simulink model "Simulation_6DOFTesting"  (R2024a)
settings: Solver=ode4  StartTime=initial_time  StopTime=final_time  FixedStep=timestep  RelTol=1e-3
values from neighbouring files (symbols this model uses):
  aEarth = 0    [CodeTesting_6DOF.m]    (also in Constants_6DOF.m = 6378137; Constants_6DOFTesting.m = 6378137)
  alphaArray = [-30, -25, -20, -15, -10, -5, 0, 5, 10, 15, 20, 25, 30]    [CodeTesting_6DOF.m]    (also in Constants_6DOF.m; Constants_6DOFTesting.m)
  altitudeArray = [0, 1000, 2000, 3000, 4000, 5000, 6000, 7000, 8000, 9000, 10000, 15000, 20000,      25000, 30000, 35000, 40000, 45000, 50000, 55000, 60000]    [CodeTesting_6DOF.m]    (also in Constants_6DOF.m; Constants_6DOFTesting.m)
  bEarth = 0    [CodeTesting_6DOF.m]    (also in Constants_6DOF.m = 6356752.3; Constants_6DOFTesting.m = 6356752.3)
  cD_3DArray = zeros(numAoAs, numMachs, numAltitudes)    [CodeTesting_6DOF.m]    (also in Constants_6DOF.m; Constants_6DOFTesting.m)
  cL_3DArray = zeros(numAoAs, numMachs, numAltitudes)    [CodeTesting_6DOF.m]    (also in Constants_6DOF.m; Constants_6DOFTesting.m)
  densityList = rhoList    [CodeTesting_6DOF.m]    (also in Constants_6DOF.m = usAtmosphere.x_; Constants_6DOFTesting.m = usAtmosphere.x_)
  height0 = 0    [Constants_6DOF.m]    (also in Constants_6DOFTesting.m = 5000)
  heightsList = usAtmosphere.Z    [CodeTesting_6DOF.m]    (also in Constants_6DOF.m; Constants_6DOFTesting.m)
  inertialPitch0 = deg2rad(inertialPitch0)    [Constants_6DOFTesting.m]
  inertialRoll0 = deg2rad(inertialRoll0)    [Constants_6DOFTesting.m]
  inertialYaw0 = deg2rad(inertialYaw0)    [Constants_6DOFTesting.m]
  Ixx = 10    [CodeTesting_6DOF.m]    (also in Constants_6DOF.m; Constants_6DOFTesting.m = 4.88094462)
  Ixz = 10    [CodeTesting_6DOF.m]    (also in Constants_6DOF.m = 1; Constants_6DOFTesting.m = 4.88094462)
  Iyy = 10    [CodeTesting_6DOF.m]    (also in Constants_6DOF.m; Constants_6DOFTesting.m = 4.88094462)
  Izz = 10    [CodeTesting_6DOF.m]    (also in Constants_6DOF.m; Constants_6DOFTesting.m = 4.88094462)
  latitude0 = pi/4    (= 0.785398163397)    [CodeTesting_6DOF.m]    (also in Constants_6DOF.m = deg2rad(latitude0); Constants_6DOFTesting.m = deg2rad(latitude0))
  longitude0 = pi/4    (= 0.785398163397)    [CodeTesting_6DOF.m]    (also in Constants_6DOF.m = deg2rad(longitude0); Constants_6DOFTesting.m = deg2rad(longitude0))
  m0 = 10    [CodeTesting_6DOF.m]    (also in Constants_6DOF.m = 50; Constants_6DOFTesting.m = 14.5939029)
  machArray = [0.5, 1.0, 1.5, 2.0, 2.5, 3.0, 3.5, 4.0, 4.5, 5.0, 5.5, 6.0, 6.5, 7.0, 7.5, 8.0,      8.5, 9.0, 9.5, 10.0]    [CodeTesting_6DOF.m]    (also in Constants_6DOF.m; Constants_6DOFTesting.m)
  omegaEarth = omega_earth    (= 7.2921159e-05)    [CodeTesting_6DOF.m]    (also in Constants_6DOF.m; Constants_6DOFTesting.m)
  p0Body = deg2rad(p0Body)    [Constants_6DOFTesting.m]
  phiBody0 = deg2rad(phiBody0)    [Constants_6DOFTesting.m]
  psiBody0 = deg2rad(psiBody0)    [Constants_6DOFTesting.m]
  q0Body = deg2rad(q0Body)    [Constants_6DOFTesting.m]
  r0Body = deg2rad(r0Body)    [Constants_6DOFTesting.m]
  rEarth = r_earth    (= 6371008.8)    [CodeTesting_6DOF.m]    (also in Constants_6DOF.m; Constants_6DOFTesting.m)
  temperatureList = usAtmosphere.T    [CodeTesting_6DOF.m]    (also in Constants_6DOF.m; Constants_6DOFTesting.m)
  thetaBody0 = deg2rad(thetaBody0)    [Constants_6DOFTesting.m]
  u0Body = 304.8    [Constants_6DOFTesting.m]
  v0Body = 0    [Constants_6DOFTesting.m]
  w0Body = -1 * w0Body    (= 0)    [Constants_6DOFTesting.m]
  wingArea = 0    [CodeTesting_6DOF.m]    (also in Constants_6DOF.m = 50; Constants_6DOFTesting.m = 0.09290304)
undefined symbols (not defined in the file or in its folder): inertialX0, inertialY0, inertialZ0
libraries: simulink_extras x18
(part 1 of 2)
settings Model: Creator=641893  LastModifiedBy=641893

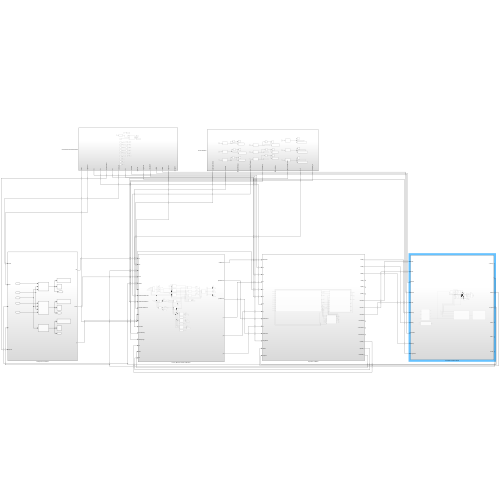
[thumbnail: Simulink's stored preview of the top-level diagram]
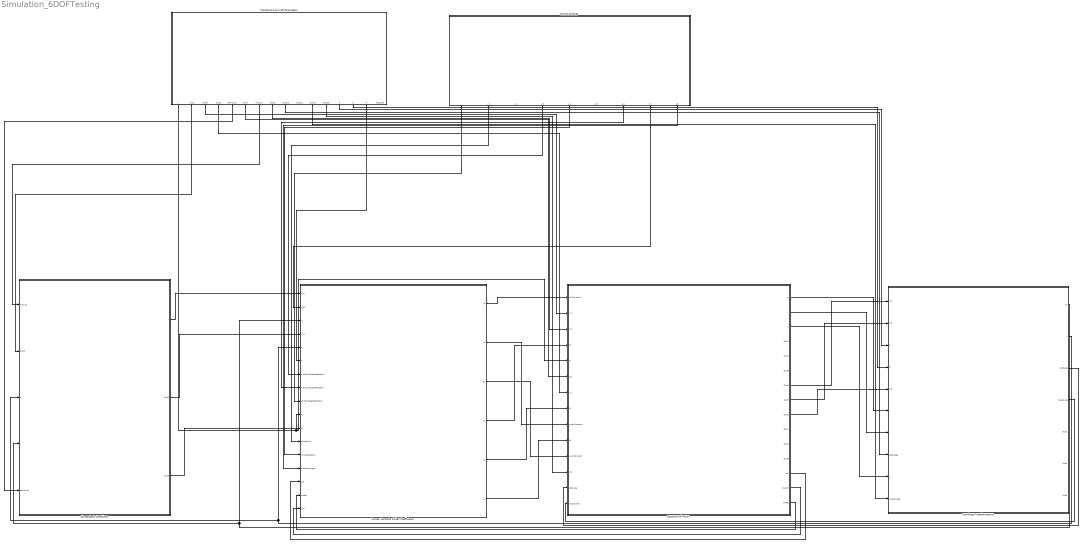
== system Simulation_6DOFTesting ==
  Atmospheric Conditions : Subsystem
  Constants & Aircraft Parameters : Subsystem
  Control Surfaces : Subsystem
  Coordinate Transformations : Subsystem
  Equations of Motion : Subsystem
  "Forces, Moments & their Coefficients" : Subsystem
  wires:
  Atmospheric Conditions/1(y) -> "Forces, Moments & their Coefficients"/1(rho)
  Atmospheric Conditions/2(Out2) -> "Forces, Moments & their Coefficients"/4(In4)
  Atmospheric Conditions/3(Out3) -> "Forces, Moments & their Coefficients"/11(g)
  Constants & Aircraft Parameters/7(rhoList) -> Atmospheric Conditions/1(rhoList)
  Constants & Aircraft Parameters/2(hList) -> Atmospheric Conditions/2(hList)
  Constants & Aircraft Parameters/5(tempList) -> Atmospheric Conditions/5(tempList)
  Coordinate Transformations/1(y4) -> "Forces, Moments & their Coefficients"/3(v), Atmospheric Conditions/4(v)
  Coordinate Transformations/2(y) -> "Forces, Moments & their Coefficients"/5(y), Atmospheric Conditions/3(r)
  Constants & Aircraft Parameters/15(A) -> "Forces, Moments & their Coefficients"/6(A)
  Constants & Aircraft Parameters/1(y) -> Equations of Motion/5(m), "Forces, Moments & their Coefficients"/10(m)
  Control Surfaces/1(y) -> "Forces, Moments & their Coefficients"/9(rollSurfaceDeflection)
  Control Surfaces/4(y3) -> "Forces, Moments & their Coefficients"/7(pitchSurfaceDeflection)
  Control Surfaces/7(y6) -> "Forces, Moments & their Coefficients"/8(yawSurfaceDeflection)
  Control Surfaces/2(y1) -> "Forces, Moments & their Coefficients"/12(thrustAoA)
  Control Surfaces/5(y4) -> "Forces, Moments & their Coefficients"/13(thrustSideslip)
  "Forces, Moments & their Coefficients"/1(y5) -> Equations of Motion/1(rollMoment)
  "Forces, Moments & their Coefficients"/2(y8) -> Equations of Motion/9(pitchMoment)
  "Forces, Moments & their Coefficients"/3(y11) -> Equations of Motion/11(yawMoment)
  "Forces, Moments & their Coefficients"/6(y3) -> Equations of Motion/10(Fz)
  "Forces, Moments & their Coefficients"/5(y2) -> Equations of Motion/8(Fy)
  "Forces, Moments & their Coefficients"/4(y1) -> Equations of Motion/4(Fx)
  Constants & Aircraft Parameters/3(Out4) -> Equations of Motion/2(Ixx)
  Constants & Aircraft Parameters/4(Out5) -> Equations of Motion/7(Iyy)
  Constants & Aircraft Parameters/6(Out7) -> Equations of Motion/6(Izz)
  Constants & Aircraft Parameters/8(Out9) -> Equations of Motion/3(Ixz)
  Equations of Motion/1(u) -> Coordinate Transformations/6(u)
  Equations of Motion/2(v) -> Coordinate Transformations/7(v)
  Equations of Motion/3(w) -> Coordinate Transformations/9(w)
  Constants & Aircraft Parameters/9(Out10) -> Coordinate Transformations/8(latitude0)
  Constants & Aircraft Parameters/13(a) -> Coordinate Transformations/3(a)
  Constants & Aircraft Parameters/14(b) -> Coordinate Transformations/4(b)
  Constants & Aircraft Parameters/11(Out12) -> Coordinate Transformations/10(longitude0)
  Equations of Motion/7(Out4) -> Coordinate Transformations/1(In1)
  Equations of Motion/8(Out5) -> Coordinate Transformations/2(In3)
  Equations of Motion/9(Out6) -> Coordinate Transformations/5(In8)
  Control Surfaces/8(y7) -> "Forces, Moments & their Coefficients"/2(AoA)
  Control Surfaces/9(y8) -> "Forces, Moments & their Coefficients"/14(sideslipAngle)
  Equations of Motion/13(phi) -> "Forces, Moments & their Coefficients"/15(psi)
  Equations of Motion/15(theta) -> "Forces, Moments & their Coefficients"/16(theta)
  Equations of Motion/14(Out10) -> "Forces, Moments & their Coefficients"/17(phi)
  Constants & Aircraft Parameters/12(Out13) -> Equations of Motion/12(In1)
  Coordinate Transformations/3(latitude) -> Equations of Motion/13(latitude)
  Coordinate Transformations/4(longitude) -> Equations of Motion/14(longitude)

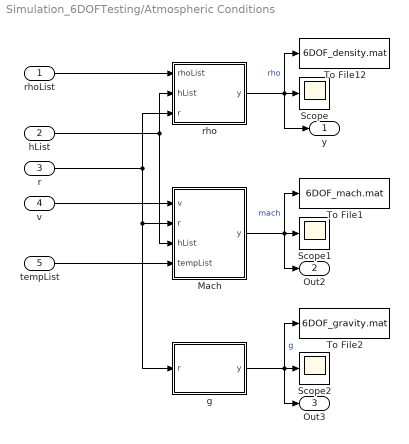
== system Simulation_6DOFTesting/Atmospheric Conditions ==
  rhoList : Inport
  hList : Inport  Port=2
  r : Inport  Port=3
  v : Inport  Port=4
  tempList : Inport  Port=5
  Mach : MATLAB Function  TreatAsAtomicUnit=on
  Scope : Scope
  Scope1 : Scope
  Scope2 : Scope
  To File1 : ToFile  Filename=6DOF_mach.mat
  To File12 : ToFile  Filename=6DOF_density.mat
  To File2 : ToFile  Filename=6DOF_gravity.mat
  g : MATLAB Function  TreatAsAtomicUnit=on
  rho : MATLAB Function  TreatAsAtomicUnit=on
  y : Outport
  Out2 : Outport  Port=2
  Out3 : Outport  Port=3
  wires:
  rho/1(y) -> Scope/1, To File12/1, y/1  "rho"
  Mach/1(y) -> Scope1/1, To File1/1, Out2/1  "mach"
  g/1(y) -> To File2/1, Scope2/1, Out3/1  "g"
  hList/1 -> rho/2(hList), Mach/3(hList)
  v/1 -> Mach/1(v)
  tempList/1 -> Mach/4(tempList)
  r/1 -> rho/3(r), g/1(r), Mach/2(r)
  rhoList/1 -> rho/1(rhoList)

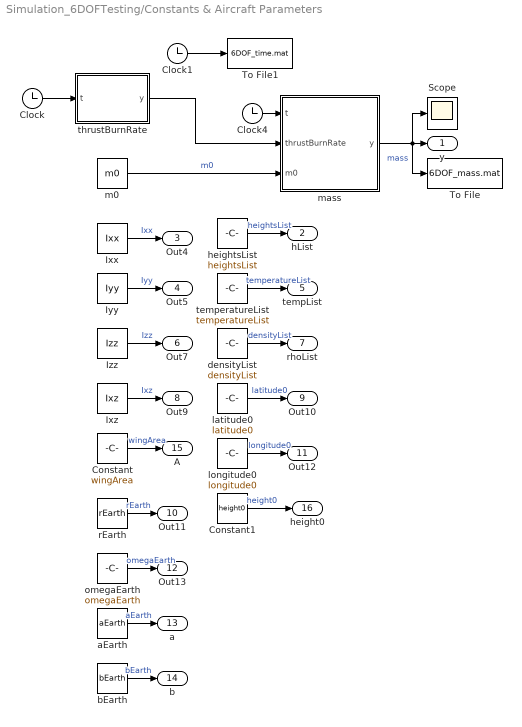
== system Simulation_6DOFTesting/Constants & Aircraft Parameters ==
  Clock : Clock
  Clock1 : Clock
  Clock4 : Clock
  Constant : Constant  Value=wingArea
  Constant1 : Constant  Value=height0
  Ixx : Constant  Value=Ixx
  Ixz : Constant  Value=Ixz
  Iyy : Constant  Value=Iyy
  Izz : Constant  Value=Izz
  Scope : Scope
  To File : ToFile  Filename=6DOF_mass.mat
  To File1 : ToFile  Filename=6DOF_time.mat
  aEarth : Constant  Value=aEarth
  bEarth : Constant  Value=bEarth
  densityList : Constant  Value=densityList
  heightsList : Constant  Value=heightsList
  latitude0 : Constant  Value=latitude0
  longitude0 : Constant  Value=longitude0
  m0 : Constant  Value=m0
  mass : MATLAB Function  TreatAsAtomicUnit=on
  omegaEarth : Constant  Value=omegaEarth
  rEarth : Constant  Value=rEarth
  temperatureList : Constant  Value=temperatureList
  thrustBurnRate : MATLAB Function  TreatAsAtomicUnit=on
  y : Outport
  hList : Outport  Port=2
  Out4 : Outport  Port=3
  Out5 : Outport  Port=4
  tempList : Outport  Port=5
  Out7 : Outport  Port=6
  rhoList : Outport  Port=7
  Out9 : Outport  Port=8
  Out10 : Outport  Port=9
  Out11 : Outport  Port=10
  Out12 : Outport  Port=11
  Out13 : Outport  Port=12
  a : Outport  Port=13
  b : Outport  Port=14
  A : Outport  Port=15
  height0 : Outport  Port=16
  wires:
  m0/1 -> mass/3(m0)  "m0"
  Clock4/1 -> mass/1(t)
  heightsList/1 -> hList/1  "heightsList"
  Clock/1 -> thrustBurnRate/1(t)
  omegaEarth/1 -> Out13/1  "omegaEarth"
  thrustBurnRate/1(y) -> mass/2(thrustBurnRate)
  rEarth/1 -> Out11/1  "rEarth"
  latitude0/1 -> Out10/1  "latitude0"
  mass/1(y) -> To File/1, Scope/1, y/1  "mass"
  aEarth/1 -> a/1  "aEarth"
  densityList/1 -> rhoList/1  "densityList"
  longitude0/1 -> Out12/1  "longitude0"
  bEarth/1 -> b/1  "bEarth"
  Izz/1 -> Out7/1  "Izz"
  Ixz/1 -> Out9/1  "Ixz"
  Ixx/1 -> Out4/1  "Ixx"
  temperatureList/1 -> tempList/1  "temperatureList"
  Iyy/1 -> Out5/1  "Iyy"
  Constant/1 -> A/1  "wingArea"
  Clock1/1 -> To File1/1
  Constant1/1 -> height0/1  "height0"

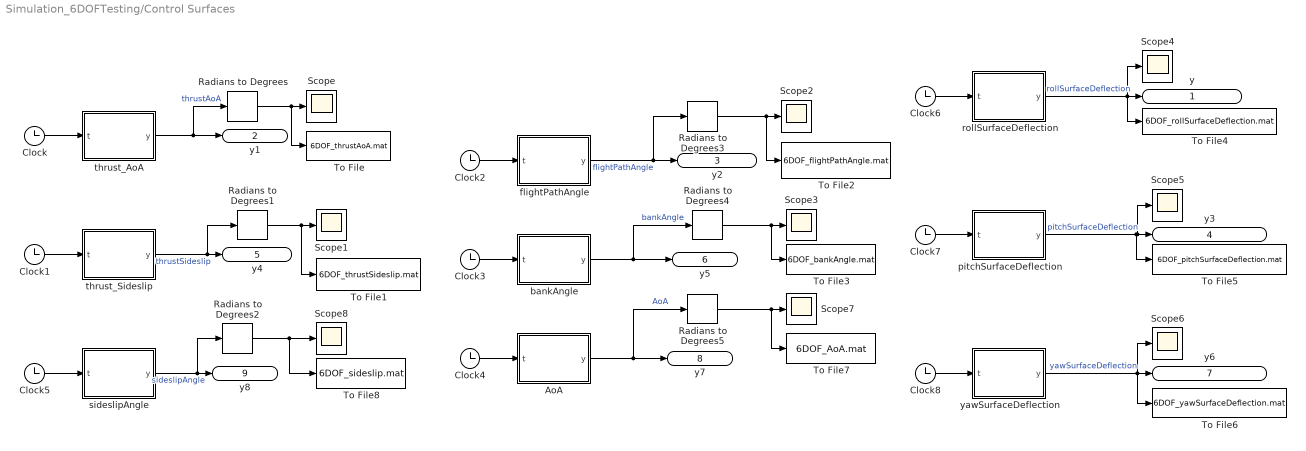
== system Simulation_6DOFTesting/Control Surfaces ==
  AoA : MATLAB Function  TreatAsAtomicUnit=on
  Clock{,1..8} (9 alike) : Clock
  Radians to Degrees{,1..5} (6 alike) : simulink_extras/Transformations/Radians to Degrees
  Scope{,1..8} (9 alike) : Scope
  To File : ToFile  Filename=6DOF_thrustAoA.mat
  To File1 : ToFile  Filename=6DOF_thrustSideslip.mat
  To File2 : ToFile  Filename=6DOF_flightPathAngle.mat
  To File3 : ToFile  Filename=6DOF_bankAngle.mat
  To File4 : ToFile  Filename=6DOF_rollSurfaceDeflection.mat
  To File5 : ToFile  Filename=6DOF_pitchSurfaceDeflection.mat
  To File6 : ToFile  Filename=6DOF_yawSurfaceDeflection.mat
  To File7 : ToFile  Filename=6DOF_AoA.mat
  To File8 : ToFile  Filename=6DOF_sideslip.mat
  bankAngle : MATLAB Function  TreatAsAtomicUnit=on
  flightPathAngle : MATLAB Function  TreatAsAtomicUnit=on
  pitchSurfaceDeflection : MATLAB Function  TreatAsAtomicUnit=on
  rollSurfaceDeflection : MATLAB Function  TreatAsAtomicUnit=on
  sideslipAngle : MATLAB Function  TreatAsAtomicUnit=on
  thrust_AoA : MATLAB Function  TreatAsAtomicUnit=on
  thrust_Sideslip : MATLAB Function  TreatAsAtomicUnit=on
  yawSurfaceDeflection : MATLAB Function  TreatAsAtomicUnit=on
  y : Outport
  y1 : Outport  Port=2
  y2 : Outport  Port=3
  y3 : Outport  Port=4
  y4 : Outport  Port=5
  y5 : Outport  Port=6
  y6 : Outport  Port=7
  y7 : Outport  Port=8
  y8 : Outport  Port=9
  wires:
  Clock8/1 -> yawSurfaceDeflection/1(t)
  rollSurfaceDeflection/1(y) -> Scope4/1, y/1, To File4/1  "rollSurfaceDeflection"
  Clock1/1 -> thrust_Sideslip/1(t)
  bankAngle/1(y) -> Radians to Degrees4/1, y5/1  "bankAngle"
  Clock6/1 -> rollSurfaceDeflection/1(t)
  Clock7/1 -> pitchSurfaceDeflection/1(t)
  pitchSurfaceDeflection/1(y) -> To File5/1, Scope5/1, y3/1  "pitchSurfaceDeflection"
  Clock2/1 -> flightPathAngle/1(t)
  thrust_AoA/1(y) -> Radians to Degrees/1, y1/1  "thrustAoA"
  Clock/1 -> thrust_AoA/1(t)
  Clock3/1 -> bankAngle/1(t)
  thrust_Sideslip/1(y) -> Radians to Degrees1/1, y4/1  "thrustSideslip"
  flightPathAngle/1(y) -> Radians to Degrees3/1, y2/1  "flightPathAngle"
  yawSurfaceDeflection/1(y) -> Scope6/1, y6/1, To File6/1  "yawSurfaceDeflection"
  AoA/1(y) -> Radians to Degrees5/1, y7/1  "AoA"
  Clock4/1 -> AoA/1(t)
  sideslipAngle/1(y) -> Radians to Degrees2/1, y8/1  "sideslipAngle"
  Clock5/1 -> sideslipAngle/1(t)
  Radians to Degrees/1 -> To File/1, Scope/1
  Radians to Degrees1/1 -> To File1/1, Scope1/1
  Radians to Degrees2/1 -> To File8/1, Scope8/1
  Radians to Degrees3/1 -> To File2/1, Scope2/1
  Radians to Degrees4/1 -> Scope3/1, To File3/1
  Radians to Degrees5/1 -> Scope7/1, To File7/1

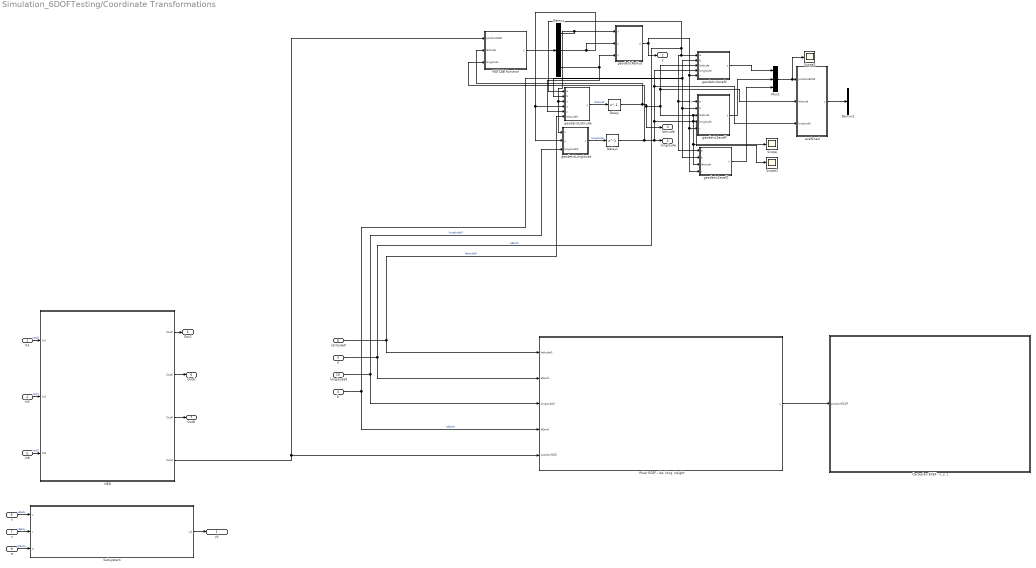
== system Simulation_6DOFTesting/Coordinate Transformations ==
  In1 : Inport
  In3 : Inport  Port=2
  a : Inport  Port=3
  b : Inport  Port=4
  In8 : Inport  Port=5
  u : Inport  Port=6
  v : Inport  Port=7
  latitude0 : Inport  Port=8
  w : Inport  Port=9
  longitude0 : Inport  Port=10
  "Cartesian ECEF - x, y, z" : Subsystem
  Delay : Delay  DelayLength=1  InitialCondition=0
  Delay1 : Delay  DelayLength=1  InitialCondition=0
  Demux : Demux  Outputs=3
  Demux1 : Demux  Outputs=3
  MATLAB Function : MATLAB Function  TreatAsAtomicUnit=on
  Mux1 : Mux  Inputs=3
  NED : Subsystem
  "Polar ECEF - lat, long, height" : Subsystem
  Scope : Scope
  Scope1 : Scope
  Scope2 : Scope
  Subsystem : Subsystem
  ecef2ned : MATLAB Function  TreatAsAtomicUnit=on
  geodetic2ecefX : MATLAB Function  TreatAsAtomicUnit=on
  geodetic2ecefY : MATLAB Function  TreatAsAtomicUnit=on
  geodetic2ecefZ : MATLAB Function  TreatAsAtomicUnit=on
  geodeticLatitude : MATLAB Function  TreatAsAtomicUnit=on
  geodeticLongitude : MATLAB Function  TreatAsAtomicUnit=on
  geodeticRadius : MATLAB Function  TreatAsAtomicUnit=on
  y4 : Outport
  y : Outport  Port=2
  latitude : Outport  Port=3
  longitude : Outport  Port=4
  Out2 : Outport  Port=5
  Out6 : Outport  Port=6
  Out8 : Outport  Port=7
  wires:
  geodeticRadius/1(y) -> geodetic2ecefX/5(r), geodetic2ecefY/5(r), geodetic2ecefZ/4(r), y/1  "r"
  ecef2ned/1(y) -> Demux1/1
  geodeticLongitude/1(y) -> Delay1/1  "longitude"
  b/1 -> "Polar ECEF - lat, long, height"/4(bEarth), geodetic2ecefX/2(b), geodeticLatitude/2(b), geodetic2ecefY/2(b), geodetic2ecefZ/2(b)  "bEarth"
  longitude0/1 -> "Polar ECEF - lat, long, height"/3(longitude0), geodeticLongitude/3(longitude0)  "longitude0"
  latitude0/1 -> geodeticLatitude/6(latitude0), "Polar ECEF - lat, long, height"/1(latitude0)  "latitude0"
  a/1 -> "Polar ECEF - lat, long, height"/2(aEarth), geodeticLatitude/1(a), geodetic2ecefX/1(a), geodetic2ecefZ/1(a), geodetic2ecefY/1(a)  "aEarth"
  geodeticLatitude/1(y) -> Delay/1  "latitude"
  Mux1/1 -> Scope2/1, ecef2ned/1(positionECEF)
  geodetic2ecefX/1(y) -> Mux1/1
  geodetic2ecefY/1(y) -> Mux1/2
  geodetic2ecefZ/1(y) -> Mux1/3
  MATLAB Function/1(y) -> Demux/1
  Demux/1 -> geodeticRadius/1(x), geodeticLatitude/3(x), geodeticLongitude/1(x)
  Demux/2 -> geodeticLongitude/2("y "), geodeticLatitude/4("y "), geodeticRadius/2("y ")
  Demux/3 -> geodeticLatitude/5(z), geodeticRadius/3(z)
  Delay/1 -> MATLAB Function/2(latitude), latitude/1, geodetic2ecefZ/3(latitude), Scope/1, geodetic2ecefY/3(latitude), geodetic2ecefX/3(latitude), ecef2ned/2(latitude)
  Delay1/1 -> MATLAB Function/3(longitude), longitude/1, Scope1/1, geodetic2ecefY/4(longitude), ecef2ned/3(longitude), geodetic2ecefX/4(longitude)
  NED/4(Out4) -> MATLAB Function/1(positionNED), "Polar ECEF - lat, long, height"/5(positionNED)
  In1/1 -> NED/1(In1)  "nedX"
  In3/1 -> NED/2(In3)  "nedY"
  In8/1 -> NED/3(In8)  "nedZ"
  NED/1(Out2) -> Out2/1
  NED/2(Out6) -> Out6/1
  NED/3(Out8) -> Out8/1
  "Polar ECEF - lat, long, height"/1(y) -> "Cartesian ECEF - x, y, z"/1(positionECEF)
  u/1 -> Subsystem/1(u)  "uBody"
  v/1 -> Subsystem/2(v)  "vBody"
  w/1 -> Subsystem/3(w)  "wBody"
  Subsystem/1(y4) -> y4/1

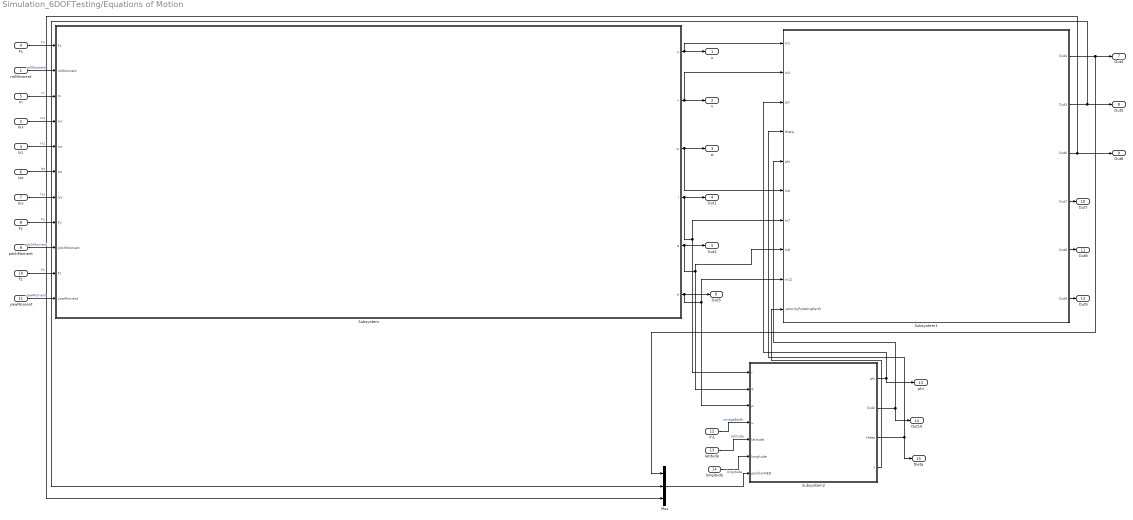
== system Simulation_6DOFTesting/Equations of Motion ==
  rollMoment : Inport
  Ixx : Inport  Port=2
  Ixz : Inport  Port=3
  Fx : Inport  Port=4
  m : Inport  Port=5
  Izz : Inport  Port=6
  Iyy : Inport  Port=7
  Fy : Inport  Port=8
  pitchMoment : Inport  Port=9
  Fz : Inport  Port=10
  yawMoment : Inport  Port=11
  In1 : Inport  Port=12
  latitude : Inport  Port=13
  longitude : Inport  Port=14
  Mux : Mux  Inputs=3
  Subsystem : Subsystem
  Subsystem1 : Subsystem
  Subsystem2 : Subsystem
  u : Outport
  v : Outport  Port=2
  w : Outport  Port=3
  Out1 : Outport  Port=4
  Out2 : Outport  Port=5
  Out3 : Outport  Port=6
  Out4 : Outport  Port=7
  Out5 : Outport  Port=8
  Out6 : Outport  Port=9
  Out7 : Outport  Port=10
  Out8 : Outport  Port=11
  Out9 : Outport  Port=12
  phi : Outport  Port=13
  Out10 : Outport  Port=14
  theta : Outport  Port=15
  wires:
  Fx/1 -> Subsystem/1(Fx)  "Fx"
  rollMoment/1 -> Subsystem/2(rollMoment)  "rollMoment"
  m/1 -> Subsystem/3(m)  "m"
  Ixx/1 -> Subsystem/4(Ixx)  "Ixx"
  Ixz/1 -> Subsystem/5(Ixz)  "Ixz"
  Izz/1 -> Subsystem/6(Izz)  "Izz"
  Iyy/1 -> Subsystem/7(Iyy)  "Iyy"
  Fy/1 -> Subsystem/8(Fy)  "Fy"
  pitchMoment/1 -> Subsystem/9(pitchMoment)  "pitchMoment"
  Fz/1 -> Subsystem/10(Fz)  "Fz"
  yawMoment/1 -> Subsystem/11(yawMoment)  "yawMoment"
  Subsystem/1(u) -> Subsystem1/1(In1), u/1
  Subsystem/2(v) -> Subsystem1/2(In2), v/1
  Subsystem/3(w) -> Subsystem1/6(In6), w/1
  Subsystem/4(r) -> Subsystem2/1(r), Subsystem1/7(In7), Out1/1
  Subsystem/5(q) -> Subsystem2/2(q), Subsystem1/8(In8), Out2/1
  Subsystem/6(p) -> Subsystem2/3(p), Subsystem1/9(In12), Out3/1
  Subsystem1/1(Out4) -> Mux/1, Out4/1
  Subsystem1/2(Out5) -> Mux/2, Out5/1
  Subsystem1/3(Out6) -> Mux/3, Out6/1
  Subsystem1/4(Out7) -> Out7/1
  Subsystem1/5(Out8) -> Out8/1
  Subsystem1/6(Out9) -> Out9/1
  Subsystem2/1(phi) -> Subsystem1/3(psi), phi/1
  Subsystem2/3(theta) -> Subsystem1/4(theta), theta/1
  Subsystem2/2(Out2) -> Subsystem1/5(phi), Out10/1
  In1/1 -> Subsystem2/4(u)  "omegaEarth"
  Subsystem2/4(y) -> Subsystem1/10(velocityRotatingEarth)
  latitude/1 -> Subsystem2/5(latitude)  "latitude"
  longitude/1 -> Subsystem2/6(longitude)  "longitude"
  Mux/1 -> Subsystem2/7(positionNED)

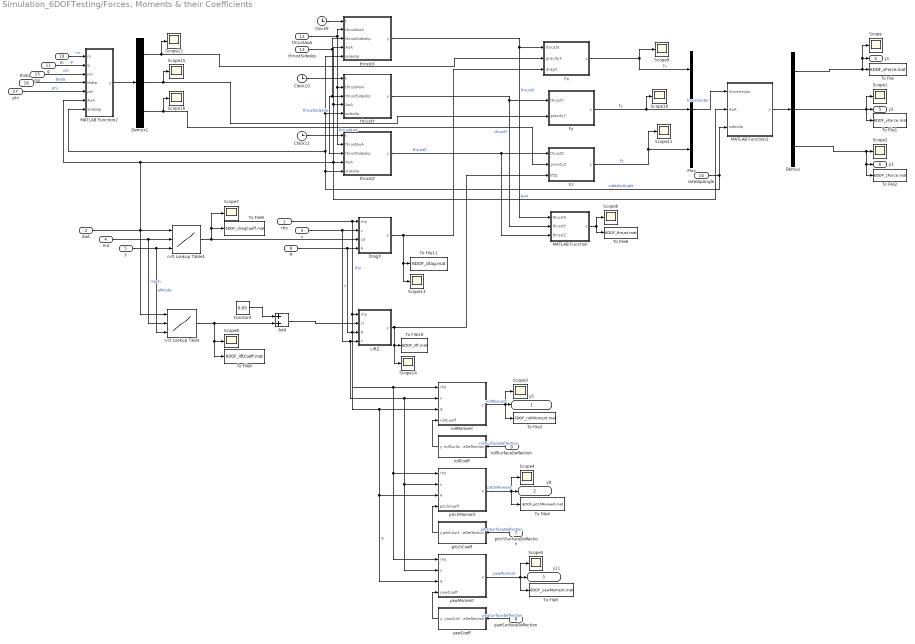
== system Simulation_6DOFTesting/Forces, Moments & their Coefficients ==
  rho : Inport
  AoA : Inport  Port=2
  v : Inport  Port=3
  In4 : Inport  Port=4
  y : Inport  Port=5
  A : Inport  Port=6
  pitchSurfaceDeflection : Inport  Port=7
  yawSurfaceDeflection : Inport  Port=8
  rollSurfaceDeflection : Inport  Port=9
  m : Inport  Port=10
  g : Inport  Port=11
  thrustAoA : Inport  Port=12
  thrustSideslip : Inport  Port=13
  sideslipAngle : Inport  Port=14
  psi : Inport  Port=15
  theta : Inport  Port=16
  phi : Inport  Port=17
  Add : Sum
  Clock10 : Clock
  Clock11 : Clock
  Clock9 : Clock
  Constant : Constant  Value=0.05
  Demux : Demux  Outputs=3
  Demux1 : Demux  Outputs=3
  DragX : MATLAB Function  TreatAsAtomicUnit=on
  Fx : MATLAB Function  TreatAsAtomicUnit=on
  Fy : MATLAB Function  TreatAsAtomicUnit=on
  Fz : MATLAB Function  TreatAsAtomicUnit=on
  LiftZ : MATLAB Function  TreatAsAtomicUnit=on
  MATLAB Function : MATLAB Function  TreatAsAtomicUnit=on
  MATLAB Function1 : MATLAB Function  TreatAsAtomicUnit=on
  MATLAB Function2 : MATLAB Function  TreatAsAtomicUnit=on
  Mux : Mux  Inputs=3
  Scope{,1..16} (17 alike) : Scope
  To File : ToFile  Filename=6DOF_xForce.mat
  To File1 : ToFile  Filename=6DOF_yForce.mat
  To File10 : ToFile  Filename=6DOF_lift.mat
  To File11 : ToFile  Filename=6DOF_drag.mat
  To File2 : ToFile  Filename=6DOF_zForce.mat
  To File3 : ToFile  Filename=6DOF_rollMoment.mat
  To File4 : ToFile  Filename=6DOF_pitchMoment.mat
  To File5 : ToFile  Filename=6DOF_yawMoment.mat
  To File6 : ToFile  Filename=6DOF_thrust.mat
  To File8 : ToFile  Filename=6DOF_liftCoeff.mat
  To File9 : ToFile  Filename=6DOF_dragCoeff.mat
  n-D Lookup Table : Lookup_n-D  NumberOfTableDimensions=3  BreakpointsForDimension1=alphaArray  BreakpointsForDimension2=machArray  BreakpointsForDimension3=altitudeArray  IndexSearchMethod=Linear search  Table=cL_3DArray  InterpMethod=Linear Lagrange  InternalRulePriority=Speed  RndMeth=Simplest
      settings: InputPortMap=u0,u1,u2
  n-D Lookup Table1 : Lookup_n-D  NumberOfTableDimensions=3  BreakpointsForDimension1=alphaArray  BreakpointsForDimension2=machArray  BreakpointsForDimension3=altitudeArray  IndexSearchMethod=Linear search  Table=cD_3DArray  InterpMethod=Linear Lagrange  InternalRulePriority=Speed  RndMeth=Simplest
      settings: InputPortMap=u0,u1,u2
  pitchCoeff : MATLAB Function  TreatAsAtomicUnit=on
  pitchMoment : MATLAB Function  TreatAsAtomicUnit=on
  rollCoeff : MATLAB Function  TreatAsAtomicUnit=on
  rollMoment : MATLAB Function  TreatAsAtomicUnit=on
  thrustX : MATLAB Function  TreatAsAtomicUnit=on
  thrustY : MATLAB Function  TreatAsAtomicUnit=on
  thrustZ : MATLAB Function  TreatAsAtomicUnit=on
  yawCoeff : MATLAB Function  TreatAsAtomicUnit=on
  yawMoment : MATLAB Function  TreatAsAtomicUnit=on
  y5 : Outport
  y8 : Outport  Port=2
  y11 : Outport  Port=3
  y1 : Outport  Port=4
  y2 : Outport  Port=5
  y3 : Outport  Port=6
  wires:
  Clock11/1 -> thrustZ/1(t)
  n-D Lookup Table/1 -> Add/2, To File8/1, Scope8/1
  LiftZ/1(y) -> Fz/3(liftZ), Scope14/1, To File10/1
  n-D Lookup Table1/1 -> Scope7/1, To File9/1, DragX/3(cd)
  v/1 -> DragX/2(v), LiftZ/4(v), rollMoment/2(v), yawMoment/2(v), pitchMoment/2(v)  "v"
  DragX/1(y) -> Fx/3(dragX), Scope13/1, To File11/1
  y/1 -> n-D Lookup Table1/3, n-D Lookup Table/3  "altitude"
  rollMoment/1(y) -> Scope3/1, y5/1, To File3/1  "rollMoment"
  yawSurfaceDeflection/1 -> yawCoeff/1(yawSurfaceDeflection)  "yawSurfaceDeflection"
  yawMoment/1(y) -> To File5/1, Scope5/1, y11/1  "yawMoment"
  Clock9/1 -> thrustX/1(t)
  rho/1 -> rollMoment/1(rho), yawMoment/1(rho), pitchMoment/1(rho), LiftZ/1(rho), DragX/1(rho)  "rho"
  Clock10/1 -> thrustY/1(t)
  rollSurfaceDeflection/1 -> rollCoeff/1(rollSurfaceDeflection)  "rollSurfaceDeflection"
  AoA/1 -> n-D Lookup Table1/1, n-D Lookup Table/1, MATLAB Function2/6(AoA), thrustZ/4(AoA), thrustX/4(AoA), thrustY/4(AoA), MATLAB Function1/2(AoA)  "AoA"
  A/1 -> DragX/4(A), rollMoment/3(A), yawMoment/3(A), pitchMoment/3(A), LiftZ/3(A)  "A"
  thrustAoA/1 -> thrustZ/2(thrustAoA), thrustY/2(thrustAoA), thrustX/2(thrustAoA)  "thrustAoA"
  In4/1 -> n-D Lookup Table1/2, n-D Lookup Table/2  "mach"
  thrustSideslip/1 -> thrustX/3(thrustSideslip), thrustZ/3(thrustSideslip), thrustY/3(thrustSideslip)  "thrustSideslip"
  pitchMoment/1(y) -> Scope4/1, y8/1, To File4/1  "pitchMoment"
  pitchSurfaceDeflection/1 -> pitchCoeff/1(pitchSurfaceDeflection)  "pitchSurfaceDeflection"
  pitchCoeff/1(y) -> pitchMoment/4(pitchCoeff)
  rollCoeff/1(y) -> rollMoment/4(rollCoeff)
  yawCoeff/1(y) -> yawMoment/4(yawCoeff)
  Fx/1(y) -> Scope9/1, Mux/1  "Fx"
  thrustX/1(y) -> MATLAB Function/1(thrustX), Fx/1(thrustX)  "thrustX"
  thrustY/1(y) -> Fy/1(thrustY), MATLAB Function/2(thrustY)  "thrustY"
  Fy/1(y) -> Scope10/1, Mux/2  "Fy"
  Fz/1(y) -> Scope11/1, Mux/3  "Fz"
  thrustZ/1(y) -> Fz/1(thrustZ), MATLAB Function/3(thrustZ)  "thrustZ"
  MATLAB Function/1(y) -> To File6/1, Scope6/1
  Add/1 -> LiftZ/2(cl)
  Constant/1 -> Add/1
  Demux/1 -> Scope/1, y1/1, To File/1
  Demux/2 -> To File1/1, y2/1, Scope1/1
  Demux/3 -> To File2/1, y3/1, Scope2/1
  Mux/1 -> MATLAB Function1/1(forceVector)  "forceVector"
  MATLAB Function1/1(y) -> Demux/1
  sideslipAngle/1 -> MATLAB Function1/3(sideslip), thrustY/5(sideslip), thrustX/5(sideslip), MATLAB Function2/7(sideslip), thrustZ/5(sideslip)  "sideslipAngle"
  Demux1/1 -> Scope12/1, Fx/2(gravityX)
  Demux1/2 -> Scope15/1, Fy/2(gravityY)
  Demux1/3 -> Scope16/1, Fz/2(gravityZ)
  MATLAB Function2/1(y) -> Demux1/1
  g/1 -> MATLAB Function2/2(g)  "g"
  m/1 -> MATLAB Function2/1(m)  "m"
  psi/1 -> MATLAB Function2/3(psi)  "psi"
  theta/1 -> MATLAB Function2/4(theta)  "theta"
  phi/1 -> MATLAB Function2/5(phi)  "phi"

== system Simulation_6DOFTesting/Coordinate Transformations/Cartesian ECEF - x, y, z ==
  positionECEF : Inport
  Demux2 : Demux  Outputs=3
  MATLAB Function : MATLAB Function  TreatAsAtomicUnit=on
  MATLAB Function4 : MATLAB Function  TreatAsAtomicUnit=on
  Scope{,2,7..8,10} (5 alike) : Scope
  To File10 : ToFile  Filename=6DOF_ecefX.mat
  To File2 : ToFile  Filename=6DOF_geodeticRadius.mat
  To File7 : ToFile  Filename=6DOF_ecefY.mat
  To File8 : ToFile  Filename=6DOF_ecefZ.mat
  wires:
  positionECEF/1 -> MATLAB Function4/1(positionECEF), MATLAB Function/1(u), Demux2/1
  Demux2/2 -> Scope7/1, To File7/1
  Demux2/3 -> To File8/1, Scope8/1
  MATLAB Function4/1(y) -> To File2/1, Scope2/1  "r"
  Demux2/1 -> Scope10/1, To File10/1
  MATLAB Function/1(y) -> Scope/1

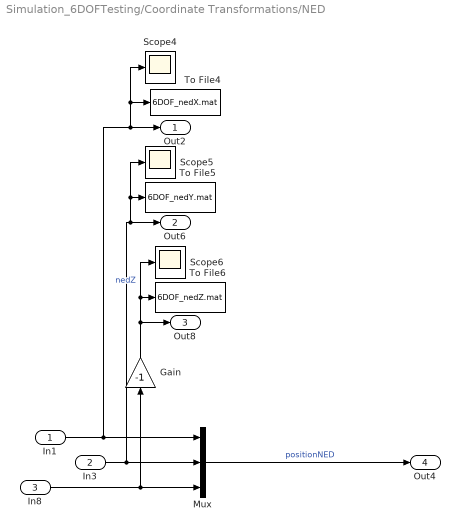
== system Simulation_6DOFTesting/Coordinate Transformations/NED ==
  In1 : Inport
  In3 : Inport  Port=2
  In8 : Inport  Port=3
  Gain : Gain  Gain=-1
  Mux : Mux  Inputs=3
  Scope4 : Scope
  Scope5 : Scope
  Scope6 : Scope
  To File4 : ToFile  Filename=6DOF_nedX.mat
  To File5 : ToFile  Filename=6DOF_nedY.mat
  To File6 : ToFile  Filename=6DOF_nedZ.mat
  Out2 : Outport
  Out6 : Outport  Port=2
  Out8 : Outport  Port=3
  Out4 : Outport  Port=4
  wires:
  In8/1 -> Mux/3, Gain/1
  In1/1 -> Out2/1, Scope4/1, To File4/1, Mux/1
  Mux/1 -> Out4/1  "positionNED"
  Gain/1 -> Out8/1, Scope6/1, To File6/1  "nedZ"
  In3/1 -> Out6/1, Scope5/1, To File5/1, Mux/2

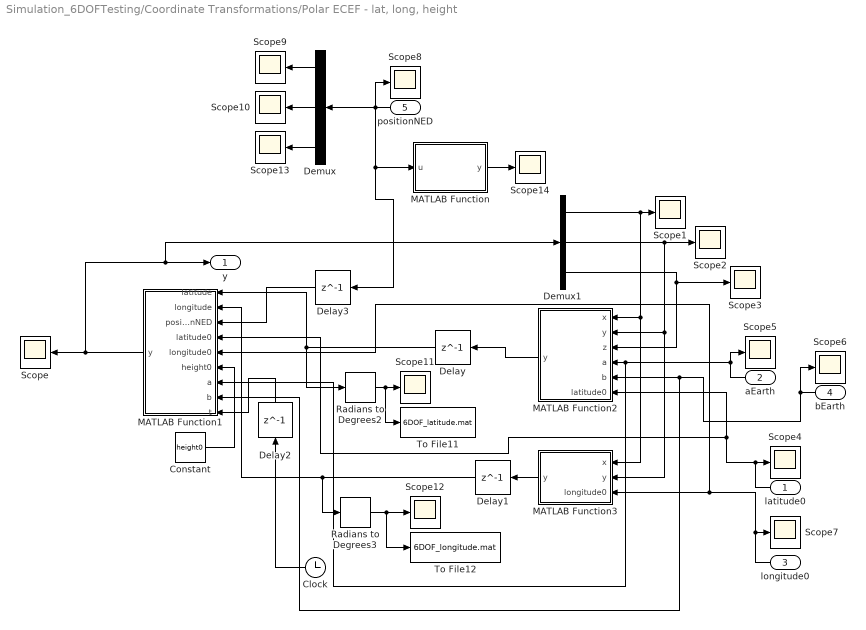
== system Simulation_6DOFTesting/Coordinate Transformations/Polar ECEF - lat, long, height ==
  latitude0 : Inport
  aEarth : Inport  Port=2
  longitude0 : Inport  Port=3
  bEarth : Inport  Port=4
  positionNED : Inport  Port=5
  Clock : Clock
  Constant : Constant  Value=height0
  Delay{,1..3} (4 alike) : Delay  DelayLength=1  InitialCondition=0
  Demux : Demux  Outputs=3
  Demux1 : Demux  Outputs=3
  MATLAB Function : MATLAB Function  TreatAsAtomicUnit=on
  MATLAB Function1 : MATLAB Function  TreatAsAtomicUnit=on
  MATLAB Function2 : MATLAB Function  TreatAsAtomicUnit=on
  MATLAB Function3 : MATLAB Function  TreatAsAtomicUnit=on
  Radians to Degrees2 : simulink_extras/Transformations/Radians to Degrees
  Radians to Degrees3 : simulink_extras/Transformations/Radians to Degrees
  Scope{,1..14} (15 alike) : Scope
  To File11 : ToFile  Filename=6DOF_latitude.mat
  To File12 : ToFile  Filename=6DOF_longitude.mat
  y : Outport
  wires:
  Radians to Degrees2/1 -> To File11/1, Scope11/1
  Radians to Degrees3/1 -> Scope12/1, To File12/1
  latitude0/1 -> MATLAB Function1/4(latitude0), MATLAB Function2/6(latitude0), Scope4/1
  bEarth/1 -> Scope6/1, MATLAB Function2/5(b), MATLAB Function1/8(b)
  MATLAB Function3/1(y) -> Delay1/1
  MATLAB Function2/1(y) -> Delay/1
  aEarth/1 -> Scope5/1, MATLAB Function1/7(a), MATLAB Function2/4(a)
  longitude0/1 -> MATLAB Function3/3(longitude0), MATLAB Function1/5(longitude0), Scope7/1
  Demux/3 -> Scope13/1
  Demux/2 -> Scope10/1
  Demux/1 -> Scope9/1
  Demux1/1 -> Scope1/1, MATLAB Function3/1(x), MATLAB Function2/1(x)
  Demux1/3 -> Scope3/1, MATLAB Function2/3(z)
  Demux1/2 -> MATLAB Function3/2("y "), MATLAB Function2/2("y "), Scope2/1
  Delay/1 -> Radians to Degrees2/1, MATLAB Function1/1(latitude)
  Delay1/1 -> MATLAB Function1/2(longitude), Radians to Degrees3/1
  positionNED/1 -> Delay3/1, MATLAB Function/1(u), Demux/1, Scope8/1
  MATLAB Function1/1(y) -> Demux1/1, y/1, Scope/1
  MATLAB Function/1(y) -> Scope14/1
  Clock/1 -> Delay2/1
  Delay2/1 -> MATLAB Function1/9(t)
  Delay3/1 -> MATLAB Function1/3(positionNED)
  Constant/1 -> MATLAB Function1/6(height0)

== system Simulation_6DOFTesting/Coordinate Transformations/Subsystem ==
  u : Inport
  v : Inport  Port=2
  w : Inport  Port=3
  Scope1 : Scope
  To File1 : ToFile  Filename=6DOF_velocity.mat
  velocity : MATLAB Function  TreatAsAtomicUnit=on
  y4 : Outport
  wires:
  v/1 -> velocity/2(v)
  velocity/1(y) -> y4/1, Scope1/1, To File1/1  "velocity"
  u/1 -> velocity/1(u)
  w/1 -> velocity/3(w)

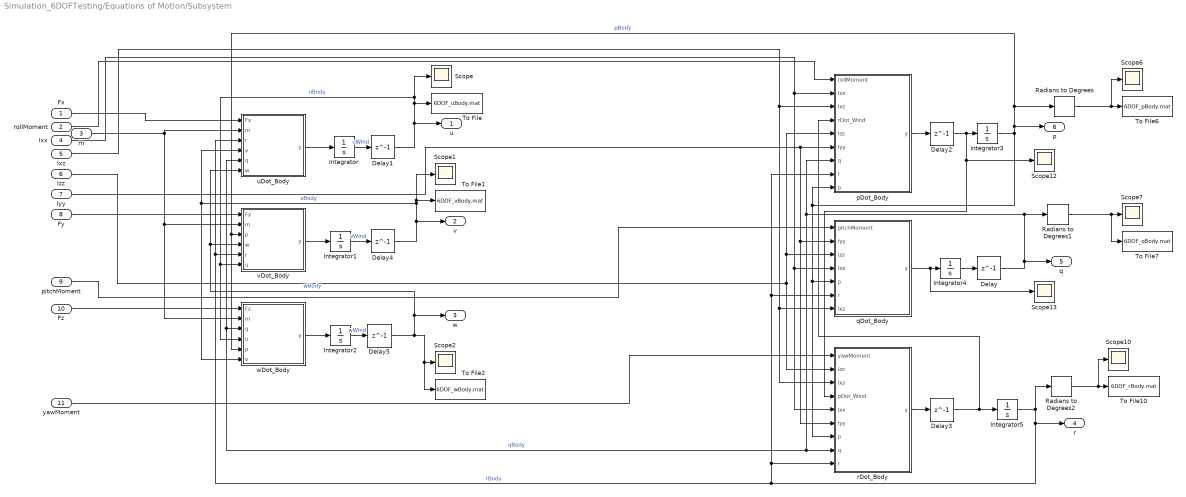
== system Simulation_6DOFTesting/Equations of Motion/Subsystem ==
  Fx : Inport
  rollMoment : Inport  Port=2
  m : Inport  Port=3
  Ixx : Inport  Port=4
  Ixz : Inport  Port=5
  Izz : Inport  Port=6
  Iyy : Inport  Port=7
  Fy : Inport  Port=8
  pitchMoment : Inport  Port=9
  Fz : Inport  Port=10
  yawMoment : Inport  Port=11
  Delay{,1..5} (6 alike) : Delay  DelayLength=1  InitialCondition=0
  Integrator : Integrator  InitialCondition=u0Body
  Integrator1 : Integrator  InitialCondition=v0Body
  Integrator2 : Integrator  InitialCondition=w0Body
  Integrator3 : Integrator  InitialCondition=p0Body
  Integrator4 : Integrator  InitialCondition=q0Body
  Integrator5 : Integrator  InitialCondition=r0Body
  Radians to Degrees : simulink_extras/Transformations/Radians to Degrees
  Radians to Degrees1 : simulink_extras/Transformations/Radians to Degrees
  Radians to Degrees2 : simulink_extras/Transformations/Radians to Degrees
  Scope{,1..2,6..7,10,12..13} (8 alike) : Scope
  To File : ToFile  Filename=6DOF_uBody.mat
  To File1 : ToFile  Filename=6DOF_vBody.mat
  To File10 : ToFile  Filename=6DOF_rBody.mat
  To File2 : ToFile  Filename=6DOF_wBody.mat
  To File6 : ToFile  Filename=6DOF_pBody.mat
  To File7 : ToFile  Filename=6DOF_qBody.mat
  pDot_Body : MATLAB Function  TreatAsAtomicUnit=on
  qDot_Body : MATLAB Function  TreatAsAtomicUnit=on
  rDot_Body : MATLAB Function  TreatAsAtomicUnit=on
  uDot_Body : MATLAB Function  TreatAsAtomicUnit=on
  vDot_Body : MATLAB Function  TreatAsAtomicUnit=on
  wDot_Body : MATLAB Function  TreatAsAtomicUnit=on
  u : Outport
  v : Outport  Port=2
  w : Outport  Port=3
  r : Outport  Port=4
  q : Outport  Port=5
  p : Outport  Port=6
  wires:
  Integrator1/1 -> Delay4/1  "vWind"
  Integrator5/1 -> Radians to Degrees2/1, r/1, vDot_Body/5(r), uDot_Body/3(r), qDot_Body/6(r), pDot_Body/8(r), rDot_Body/9(r)  "rBody"
  Fx/1 -> uDot_Body/1(Fx)
  Integrator2/1 -> Delay5/1  "wWind"
  Integrator3/1 -> p/1, Radians to Degrees/1, wDot_Body/5(p), vDot_Body/3(p), qDot_Body/5(p), rDot_Body/7(p), pDot_Body/9(p)  "pBody"
  Delay2/1 -> Scope12/1, rDot_Body/4(pDot_Wind), Integrator3/1
  uDot_Body/1(y) -> Integrator/1
  Ixx/1 -> pDot_Body/2(Ixx), qDot_Body/4(Ixx), rDot_Body/5(Ixx)
  Delay5/1 -> w/1, vDot_Body/4(w), uDot_Body/6(w), To File2/1, Scope2/1  "wBody"
  Delay1/1 -> u/1, vDot_Body/6(u), wDot_Body/4(u), Scope/1, To File/1  "uBody"
  Integrator/1 -> Delay1/1  "uWind"
  Delay3/1 -> pDot_Body/4(rDot_Wind), Integrator5/1
  Ixz/1 -> pDot_Body/3(Ixz), qDot_Body/7(Ixz), rDot_Body/3(Ixz)
  Delay4/1 -> v/1, wDot_Body/6(v), uDot_Body/4(v), Scope1/1, To File1/1  "vBody"
  pDot_Body/1(y) -> Delay2/1
  qDot_Body/1(y) -> Scope13/1, Integrator4/1
  Iyy/1 -> pDot_Body/6(Iyy), qDot_Body/2(Iyy), rDot_Body/6(Iyy)
  rDot_Body/1(y) -> Delay3/1
  wDot_Body/1(y) -> Integrator2/1
  rollMoment/1 -> pDot_Body/1(rollMoment)
  Integrator4/1 -> Delay/1
  Delay/1 -> q/1, Radians to Degrees1/1, rDot_Body/8(q), wDot_Body/3(q), uDot_Body/5(q), pDot_Body/7(q)  "qBody"
  Izz/1 -> pDot_Body/5(Izz), qDot_Body/3(Izz), rDot_Body/2(Izz)
  m/1 -> uDot_Body/2(m), vDot_Body/2(m), wDot_Body/2(m)
  vDot_Body/1(y) -> Integrator1/1
  pitchMoment/1 -> qDot_Body/1(pitchMoment)
  Fy/1 -> vDot_Body/1(Fy)
  yawMoment/1 -> rDot_Body/1(yawMoment)
  Fz/1 -> wDot_Body/1(Fz)
  Radians to Degrees/1 -> Scope6/1, To File6/1
  Radians to Degrees1/1 -> To File7/1, Scope7/1
  Radians to Degrees2/1 -> Scope10/1, To File10/1

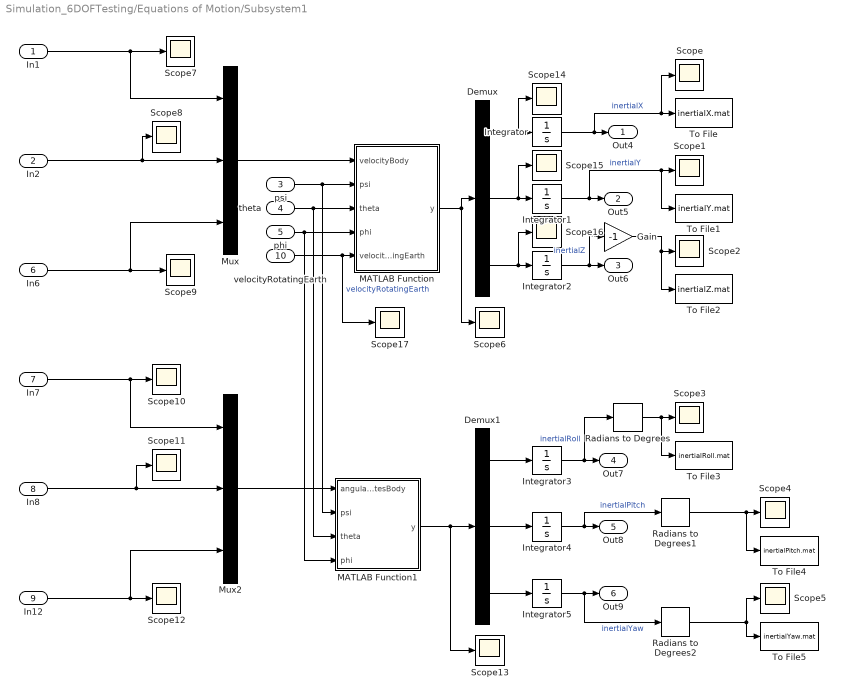
== system Simulation_6DOFTesting/Equations of Motion/Subsystem1 ==
  In1 : Inport
  In2 : Inport  Port=2
  psi : Inport  Port=3
  theta : Inport  Port=4
  phi : Inport  Port=5
  In6 : Inport  Port=6
  In7 : Inport  Port=7
  In8 : Inport  Port=8
  In12 : Inport  Port=9
  velocityRotatingEarth : Inport  Port=10
  Demux : Demux  Outputs=3
  Demux1 : Demux  Outputs=3
  Gain : Gain  Gain=-1
  Integrator : Integrator  InitialCondition=inertialX0
  Integrator1 : Integrator  InitialCondition=inertialY0
  Integrator2 : Integrator  InitialCondition=inertialZ0
  Integrator3 : Integrator  InitialCondition=inertialRoll0
  Integrator4 : Integrator  InitialCondition=inertialPitch0
  Integrator5 : Integrator  InitialCondition=inertialYaw0
  MATLAB Function : MATLAB Function  TreatAsAtomicUnit=on
  MATLAB Function1 : MATLAB Function  TreatAsAtomicUnit=on
  Mux : Mux  Inputs=3
  Mux2 : Mux  Inputs=3
  Radians to Degrees : simulink_extras/Transformations/Radians to Degrees
  Radians to Degrees1 : simulink_extras/Transformations/Radians to Degrees
  Radians to Degrees2 : simulink_extras/Transformations/Radians to Degrees
  Scope{,1..17} (18 alike) : Scope
  To File : ToFile  Filename=inertialX.mat  SaveFormat=Timeseries
  To File1 : ToFile  Filename=inertialY.mat  SaveFormat=Timeseries
  To File2 : ToFile  Filename=inertialZ.mat  SaveFormat=Timeseries
  To File3 : ToFile  Filename=inertialRoll.mat
  To File4 : ToFile  Filename=inertialPitch.mat
  To File5 : ToFile  Filename=inertialYaw.mat
  Out4 : Outport
  Out5 : Outport  Port=2
  Out6 : Outport  Port=3
  Out7 : Outport  Port=4
  Out8 : Outport  Port=5
  Out9 : Outport  Port=6
  wires:
  In6/1 -> Scope9/1, Mux/3
  Demux1/1 -> Integrator3/1
  Demux1/3 -> Integrator5/1
  Integrator4/1 -> Radians to Degrees1/1, Out8/1  "inertialPitch"
  Mux/1 -> MATLAB Function/1(velocityBody)
  Integrator/1 -> Scope/1, To File/1, Out4/1  "inertialX"
  psi/1 -> MATLAB Function1/2(psi), MATLAB Function/2(psi)
  Integrator5/1 -> Radians to Degrees2/1, Out9/1  "inertialYaw"
  Demux/1 -> Scope14/1, Integrator/1
  Demux1/2 -> Integrator4/1
  MATLAB Function/1(y) -> Scope6/1, Demux/1
  Demux/2 -> Scope15/1, Integrator1/1
  Integrator3/1 -> Radians to Degrees/1, Out7/1  "inertialRoll"
  Demux/3 -> Scope16/1, Integrator2/1
  Mux2/1 -> MATLAB Function1/1(angularRatesBody)
  In12/1 -> Mux2/3, Scope12/1
  MATLAB Function1/1(y) -> Scope13/1, Demux1/1
  Integrator2/1 -> Gain/1, Out6/1  "inertialZ"
  Integrator1/1 -> To File1/1, Scope1/1, Out5/1  "inertialY"
  In8/1 -> Scope11/1, Mux2/2
  theta/1 -> MATLAB Function1/3(theta), MATLAB Function/3(theta)
  In7/1 -> Scope10/1, Mux2/1
  In2/1 -> Scope8/1, Mux/2
  phi/1 -> MATLAB Function1/4(phi), MATLAB Function/4(phi)
  In1/1 -> Scope7/1, Mux/1
  velocityRotatingEarth/1 -> Scope17/1, MATLAB Function/5(velocityRotatingEarth)  "velocityRotatingEarth"
  Gain/1 -> To File2/1, Scope2/1
  Radians to Degrees/1 -> To File3/1, Scope3/1
  Radians to Degrees1/1 -> To File4/1, Scope4/1
  Radians to Degrees2/1 -> To File5/1, Scope5/1

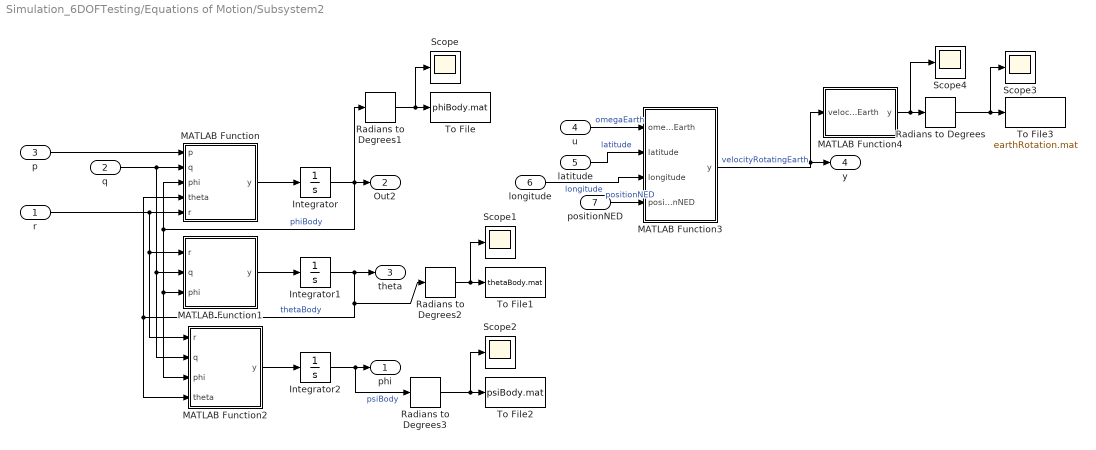
== system Simulation_6DOFTesting/Equations of Motion/Subsystem2 ==
  r : Inport
  q : Inport  Port=2
  p : Inport  Port=3
  u : Inport  Port=4
  latitude : Inport  Port=5
  longitude : Inport  Port=6
  positionNED : Inport  Port=7
  Integrator : Integrator  InitialCondition=phiBody0
  Integrator1 : Integrator  InitialCondition=thetaBody0
  Integrator2 : Integrator  InitialCondition=psiBody0
  MATLAB Function : MATLAB Function  TreatAsAtomicUnit=on
  MATLAB Function1 : MATLAB Function  TreatAsAtomicUnit=on
  MATLAB Function2 : MATLAB Function  TreatAsAtomicUnit=on
  MATLAB Function3 : MATLAB Function  TreatAsAtomicUnit=on
  MATLAB Function4 : MATLAB Function  TreatAsAtomicUnit=on
  Radians to Degrees{,1..3} (4 alike) : simulink_extras/Transformations/Radians to Degrees
  Scope{,1..4} (5 alike) : Scope
  To File : ToFile  Filename=phiBody.mat
  To File1 : ToFile  Filename=thetaBody.mat
  To File2 : ToFile  Filename=psiBody.mat
  To File3 : ToFile  Filename=earthRotation.mat
  phi : Outport
  Out2 : Outport  Port=2
  theta : Outport  Port=3
  y : Outport  Port=4
  wires:
  Integrator2/1 -> Radians to Degrees3/1, phi/1  "psiBody"
  MATLAB Function1/1(y) -> Integrator1/1
  p/1 -> MATLAB Function/1(p)
  Integrator/1 -> Radians to Degrees1/1, MATLAB Function/3(phi), MATLAB Function1/3(phi), MATLAB Function2/3(phi), Out2/1  "phiBody"
  q/1 -> MATLAB Function/2(q), MATLAB Function2/2(q), MATLAB Function1/2(q)
  MATLAB Function2/1(y) -> Integrator2/1
  r/1 -> MATLAB Function/5(r), MATLAB Function2/1(r), MATLAB Function1/1(r)
  MATLAB Function/1(y) -> Integrator/1
  Integrator1/1 -> Radians to Degrees2/1, MATLAB Function2/4(theta), MATLAB Function/4(theta), theta/1  "thetaBody"
  u/1 -> MATLAB Function3/1(omegaEarth)  "omegaEarth"
  MATLAB Function3/1(y) -> MATLAB Function4/1(velocityRotatingEarth), y/1  "velocityRotatingEarth"
  latitude/1 -> MATLAB Function3/2(latitude)  "latitude"
  longitude/1 -> MATLAB Function3/3(longitude)  "longitude"
  MATLAB Function4/1(y) -> Scope4/1, Radians to Degrees/1
  Radians to Degrees/1 -> Scope3/1, To File3/1
  Radians to Degrees1/1 -> Scope/1, To File/1
  Radians to Degrees2/1 -> Scope1/1, To File1/1
  Radians to Degrees3/1 -> Scope2/1, To File2/1
  positionNED/1 -> MATLAB Function3/4(positionNED)  "positionNED"

== matlab function Simulation_6DOFTesting/Control Surfaces/pitchSurfaceDeflection ==
  data: t input; y output
function y = fcn(t)

pitchSurfaceDeflection = 0.0;

if t > 5 && t < 15
    pitchSurfaceDeflection = 0.001;
end

if t > 20 && t < 25
    pitchSurfaceDeflection = -0.001;
end


y = pitchSurfaceDeflection;

== matlab function Simulation_6DOFTesting/Control Surfaces/yawSurfaceDeflection ==
  data: t input; y output
function y = fcn(t)

yawSurfaceDeflection = 0;

y = yawSurfaceDeflection;

== matlab function Simulation_6DOFTesting/Forces, Moments & their Coefficients/thrustX ==
  data: t input; y output; thrustAoA input; thrustSideslip input; AoA input; sideslip input
function y = fcn(t, thrustAoA, thrustSideslip, AoA, sideslip)

thrust = 0;

thrust = thrust * cos(thrustAoA) * cos(thrustSideslip);

thrustWindX = thrust * cos(AoA) * cos(sideslip);

y = thrustWindX;

== matlab function Simulation_6DOFTesting/Atmospheric Conditions/Mach ==
  data: v input; y output; r input; hList input; tempList input
function y = fcn(v, r, hList, tempList)

gamma = 1.4;
rGas = 287.05;

r = r / 10^3;

if r >= 0
    temp = interp1(hList, tempList, r);
    a = sqrt(gamma * rGas * temp);
    y = v/a;
else
    temp = 0;
    y = 0;
end

== matlab function Simulation_6DOFTesting/Forces, Moments & their Coefficients/thrustY ==
  data: t input; y output; thrustAoA input; thrustSideslip input; AoA input; sideslip input
function y = fcn(t, thrustAoA, thrustSideslip, AoA, sideslip)

thrust = 0;

thrust = thrust * cos(thrustAoA) * sin(thrustSideslip);

thrustWindY = -1 * thrust * cos(AoA) * sin(sideslip);

y = thrustWindY;

== matlab function Simulation_6DOFTesting/Forces, Moments & their Coefficients/thrustZ ==
  data: t input; y output; thrustAoA input; thrustSideslip input; AoA input; sideslip input
function y = fcn(t, thrustAoA, thrustSideslip, AoA, sideslip)

thrust = 0;

thrust = -1 * thrust * sin(thrustAoA);

thrustWindZ = -1 * thrust * sin(AoA);

y = thrustWindZ;

== matlab function Simulation_6DOFTesting/Equations of Motion/Subsystem1/MATLAB Function ==
  data: velocityBody input; y output; psi input; theta input; phi input; velocityRotatingEarth input
function y = fcn(velocityBody, psi, theta, phi, velocityRotatingEarth)

rollMatrix = [1 0 0; 0 cos(phi) -sin(phi); 0 sin(phi) cos(phi)];
pitchMatrix = [cos(theta) 0 sin(theta); 0 1 0; -sin(theta) 0 cos(theta)];
yawMatrix = [cos(psi) -sin(psi) 0; sin(psi) cos(psi) 0; 0 0 1];

rotationMatrixIB = yawMatrix * pitchMatrix * rollMatrix;

velocityInertial = (rotationMatrixIB * velocityBody) + velocityRotatingEarth;

y = velocityInertial;

== matlab function Simulation_6DOFTesting/Control Surfaces/thrust_Sideslip ==
  data: t input; y output
function y = fcn(t)

thrustSideslip = 0;

y = thrustSideslip;

== matlab function Simulation_6DOFTesting/Equations of Motion/Subsystem1/MATLAB Function1 ==
  data: angularRatesBody input; y output; psi input; theta input; phi input
function y = fcn(angularRatesBody, psi, theta, phi)

rollMatrix = [1 0 0; 0 cos(phi) -sin(phi); 0 sin(phi) cos(phi)];
pitchMatrix = [cos(theta) 0 sin(theta); 0 1 0; -sin(theta) 0 cos(theta)];
yawMatrix = [cos(psi) -sin(psi) 0; sin(psi) cos(psi) 0; 0 0 1];

rotationMatrixIB = yawMatrix * pitchMatrix * rollMatrix;

angularRatesInertial = rotationMatrixIB * angularRatesBody;

y = angularRatesInertial;

== matlab function Simulation_6DOFTesting/Equations of Motion/Subsystem2/MATLAB Function ==
  data: p input; y output; q input; phi input; theta input; r input
function y = fcn(p, q, phi, theta, r)

y = p + q * sin(phi) * tan(theta) + r * cos(phi) * tan(theta);

== matlab function Simulation_6DOFTesting/Forces, Moments & their Coefficients/rollMoment ==
  data: rho input; y output; v input; A input; rollCoeff input
function y = fcn(rho, v, A, rollCoeff)

rollMoment = 0.5 * rho * v^2 * A * rollCoeff;

y = rollMoment;

== matlab function Simulation_6DOFTesting/Forces, Moments & their Coefficients/pitchMoment ==
  data: rho input; y output; v input; A input; pitchCoeff input
function y = fcn(rho, v, A, pitchCoeff)

pitchMoment = 0.5 * rho * v^2 * A * pitchCoeff;

y = pitchMoment;

== matlab function Simulation_6DOFTesting/Forces, Moments & their Coefficients/yawMoment ==
  data: rho input; y output; v input; A input; yawCoeff input
function y = fcn(rho, v, A, yawCoeff)

yawMoment = 0.5 * rho * v^2 * A * yawCoeff;

y = yawMoment;

== matlab function Simulation_6DOFTesting/Equations of Motion/Subsystem/uDot_Body ==
  data: Fx input; y output; m input; r input; v input; q input; w input
function y = fcn(Fx, m, r, v, q, w)

uDot_Wind = (Fx/m) + r * v - q * w;

y = uDot_Wind;

== matlab function Simulation_6DOFTesting/Equations of Motion/Subsystem/vDot_Body ==
  data: Fy input; y output; m input; p input; w input; r input; u input
function y = fcn(Fy, m, p, w, r,  u)

vDot_Wind = (Fy / m) + p * w - r * u;

y = vDot_Wind;

== matlab function Simulation_6DOFTesting/Control Surfaces/thrust_AoA ==
  data: t input; y output
function y = fcn(t)

thrustAoA = 0;

y = thrustAoA;

== matlab function Simulation_6DOFTesting/Equations of Motion/Subsystem/wDot_Body ==
  data: Fz input; y output; m input; q input; u input; p input; v input
function y = fcn(Fz, m, q, u, p, v)

vDot_Wind = (Fz / m) + q * u - p * v;

y = vDot_Wind;

== matlab function Simulation_6DOFTesting/Equations of Motion/Subsystem/pDot_Body ==
  data: rollMoment input; y output; Ixx input; Ixz input; rDot_Wind input; Izz input; Iyy input; q input; r input; p input
function y = fcn(rollMoment, Ixx, Ixz, rDot_Wind, Izz, Iyy, q, r, p)

pDot_Wind = (1/Ixx) * (Ixz * rDot_Wind - (Izz - Iyy) * q * r + Ixz * p * q - rollMoment);

y = pDot_Wind;

== matlab function Simulation_6DOFTesting/Equations of Motion/Subsystem/qDot_Body ==
  data: pitchMoment input; Iyy input; Izz input; y output; Ixx input; p input; r input; Ixz input
function y = fcn(pitchMoment, Iyy, Izz, Ixx, p, r, Ixz)

pDot_Wind = (1/Iyy) * ( (Izz - Ixx) * p * r + Ixz * (p^2 - r^2) - pitchMoment);

y = pDot_Wind;

== matlab function Simulation_6DOFTesting/Equations of Motion/Subsystem/rDot_Body ==
  data: yawMoment input; Izz input; Ixz input; pDot_Wind input; y output; Ixx input; Iyy input; p input; q input; r input
function y = fcn(yawMoment, Izz, Ixz, pDot_Wind, Ixx, Iyy, p, q, r)

rDot_Wind = (1/Izz) * (Ixz * pDot_Wind - (Ixx - Iyy) * p * q + Ixz * q * r - yawMoment);

y = rDot_Wind;

== matlab function Simulation_6DOFTesting/Constants & Aircraft Parameters/mass ==
  data: t input; y output; thrustBurnRate input; m0 input
function y = fcn(t, thrustBurnRate, m0)

mass = m0 - thrustBurnRate * t;

y = mass;

== matlab function Simulation_6DOFTesting/Control Surfaces/flightPathAngle ==
  data: t input; y output
function y = fcn(t)

flightPathAngle = 0;

y = flightPathAngle;

== matlab function Simulation_6DOFTesting/Coordinate Transformations/geodeticRadius ==
  data: x input; y output; y input; z input
function y = fcn(x, y, z)

radiusGeodetic = sqrt(x^2 + y^2 + z^2);

y = radiusGeodetic;

== matlab function Simulation_6DOFTesting/Coordinate Transformations/geodeticLatitude ==
  data: a input; b input; x input; y input; z input; y output; latitude0 input
function y = fcn(a, b, x, y, z, latitude0)

latitude = atan( (a^2/b^2) * z / sqrt(x^2 + y^2) ) + latitude0;

latitude = atan( (a^2 * (sin(latitude0)^2)) / (b^2 * sin(latitude) * cos(latitude) + (sqrt(x^2 + y^2) * sin(latitude) - z * cos(latitude)) * sqrt(a^2 * (cos(latitude))^2 + b^2 * sin(latitude)^2)));

y = latitude;

== matlab function Simulation_6DOFTesting/Coordinate Transformations/geodeticLongitude ==
  data: x input; y output; y input; longitude0 input
function y = fcn(x, y, longitude0)

longitude = atan2(y,x) + longitude0;

y = longitude;

== matlab function Simulation_6DOFTesting/Coordinate Transformations/geodetic2ecefX ==
  data: a input; y output; b input; latitude input; longitude input; r input
function y = fcn(a, b, latitude, longitude, r)

rEarth = 6371.0088 * 10^3;

e = sqrt(1 - b^2/a^2);
nPhi = a / sqrt(1 - e^2 * (sin(latitude))^2);

ecefX = (nPhi + r) * cos(latitude) * cos(longitude);

y = ecefX;

== matlab function Simulation_6DOFTesting/Coordinate Transformations/geodetic2ecefY ==
  data: a input; y output; b input; latitude input; longitude input; r input
function y = fcn(a, b, latitude, longitude, r)

e = sqrt(1 - b^2/a^2);
nPhi = a / sqrt(1 - e^2 * (sin(latitude))^2);

ecefY = (nPhi + r) * cos(latitude) * sin(longitude);

y = ecefY;

== matlab function Simulation_6DOFTesting/Coordinate Transformations/geodetic2ecefZ ==
  data: a input; y output; b input; latitude input; r input
function y = fcn(a, b, latitude, r)

e = sqrt(1 - b^2/a^2);
nPhi = a / sqrt(1 - e^2 * (sin(latitude))^2);

ecefZ = ((1 - e^2) * nPhi + r) * sin(latitude);

y = ecefZ;

== matlab function Simulation_6DOFTesting/Coordinate Transformations/ecef2ned ==
  data: positionECEF input; y output; latitude input; longitude input
function y = fcn(positionECEF, latitude, longitude)

rotationMatrix = [-sin(latitude) * cos(longitude) -sin(latitude) * sin(longitude) cos(latitude); -sin(longitude) cos(longitude) 0; -cos(latitude) * cos(longitude) -cos(latitude) * sin(longitude) sin(latitude)];

nedPosition = rotationMatrix * positionECEF;

y = nedPosition;

== matlab function Simulation_6DOFTesting/Control Surfaces/bankAngle ==
  data: t input; y output
function y = fcn(t)

bankAngle = 0;

y = bankAngle;

== matlab function Simulation_6DOFTesting/Forces, Moments & their Coefficients/rollCoeff ==
  data: rollSurfaceDeflection input; y output
function y = fcn(rollSurfaceDeflection)

rollCoeff = rollSurfaceDeflection;

y = rollCoeff;

== matlab function Simulation_6DOFTesting/Forces, Moments & their Coefficients/pitchCoeff ==
  data: pitchSurfaceDeflection input; y output
function y = fcn(pitchSurfaceDeflection)

pitchCoeff = pitchSurfaceDeflection;

y = pitchCoeff;

== matlab function Simulation_6DOFTesting/Forces, Moments & their Coefficients/yawCoeff ==
  data: yawSurfaceDeflection input; y output
function y = fcn(yawSurfaceDeflection)

yawCoeff = yawSurfaceDeflection;

y = yawCoeff;

== matlab function Simulation_6DOFTesting/Constants & Aircraft Parameters/thrustBurnRate ==
  data: t input; y output
function y = fcn(t)

thrustBurnRate = 0;

y = thrustBurnRate;

== matlab function Simulation_6DOFTesting/Forces, Moments & their Coefficients/Fx ==
  data: thrustX input; y output; gravityX input; dragX input
function y = fcn(thrustX, gravityX, dragX)

xForce = thrustX + gravityX - dragX;

y = xForce;

== matlab function Simulation_6DOFTesting/Forces, Moments & their Coefficients/Fy ==
  data: thrustY input; y output; gravityY input
function y = fcn(thrustY, gravityY)

yForce = thrustY + gravityY;

y = yForce;

== matlab function Simulation_6DOFTesting/Forces, Moments & their Coefficients/Fz ==
  data: thrustZ input; y output; gravityZ input; liftZ input
function y = fcn(thrustZ, gravityZ, liftZ)

zForce = thrustZ + gravityZ - liftZ;

y = zForce;

== matlab function Simulation_6DOFTesting/Forces, Moments & their Coefficients/MATLAB Function ==
  data: thrustX input; y output; thrustY input; thrustZ input
function y = fcn(thrustX, thrustY, thrustZ)

thrustMagnitude = sqrt(thrustX^2 + thrustY^2 + thrustZ^2);

y = thrustMagnitude;

== matlab function Simulation_6DOFTesting/Forces, Moments & their Coefficients/MATLAB Function1 ==
  data: forceVector input; y output; AoA input; sideslip input
function y = fcn(forceVector, AoA, sideslip)

rotationMatrix = [cos(AoA) * cos(sideslip) -cos(AoA) * sin(sideslip) -sin(AoA); sin(sideslip) cos(sideslip) 0; sin(AoA) * cos(sideslip) -sin(AoA) * sin(sideslip) cos(AoA)];

rotatedForceVector = rotationMatrix * forceVector;

y = rotatedForceVector;

== matlab function Simulation_6DOFTesting/Coordinate Transformations/Subsystem/velocity ==
  data: u input; y output; v input; w input
function y = fcn(u, v, w)

velocity = sqrt(u^2 + v^2 + w^2);

y = velocity;

== matlab function Simulation_6DOFTesting/Forces, Moments & their Coefficients/MATLAB Function2 ==
  data: m input; g input; psi input; theta input; phi input; AoA input; y output; sideslip input
function y = fcn(m, g, psi, theta, phi, AoA, sideslip)

inertialGravity = [0; 0; m * g];

rollMatrix = [1 0 0; 0 cos(phi) -sin(phi); 0 sin(phi) cos(phi)];
pitchMatrix = [cos(theta) 0 sin(theta); 0 1 0; -sin(theta) 0 cos(theta)];
yawMatrix = [cos(psi) -sin(psi) 0; sin(psi) cos(psi) 0; 0 0 1];

rotationMatrixIB = yawMatrix * pitchMatrix * rollMatrix;

rotationBI = inv(rotationMatrixIB);
rotationWB = [cos(AoA) * cos(sideslip) -cos(AoA) * sin(sideslip) -sin(AoA); sin(sideslip) cos(sideslip) 0; sin(AoA) * cos(sideslip) -sin(AoA) * sin(sideslip) cos(AoA)];

bodyGravity = rotationBI * inertialGravity;
windGravity = rotationWB * bodyGravity;

y = windGravity;
